simulink model "rotpentemplate"  (R2021b)
settings: Solver=VariableStepDiscrete  StartTime=0.0  StopTime=50  RelTol=1e-3  EnableMultiTasking=on
values from neighbouring files (symbols this model uses):
  adingain = [adingain 1 1 1 1 1]    [hwinit.m]    (also in theta2_bottomswing.mat = [1.276 1.276 1 1 1 1 1])
  adinoffs = [adinoffs 0 0 0 0 0]    [hwinit.m]    (also in theta2_bottomswing.mat = [-3.773 -1.223 0 0 0 0 0])
  daoutgain = 1*[-6]    [hwinit.m]    (also in theta2_bottomswing.mat = -6)
  daoutoffs = [0.00]    [hwinit.m]    (also in theta2_bottomswing.mat = 0)
  h = 0.01    [hwinit.m]    (also in mpc_controller.m = zeros(dim.nx+dim.nu, 1); theta2_bottomswing.mat = 0.05)
  K_lqr = [K_lqr, 0, 0]    [mpc_controller.m]
  model_matrices = buildmatrices(xr, model_mpc, constraint, penalty, terminal)    [mpc_controller.m]
  sys_dis = c2d(sys_ct, h)    [mpc_controller.m]
  xr = xur(1:dim.nx)    [mpc_controller.m]
undefined symbols (not defined in the file or in its folder): DiscIntNeverNeededParam, Discrete, model_mpc, Time
libraries: simulink x11, ctrlSharedLib x5, simulink_extras x1
settings Model: Creator=rbabuska  LastModifiedBy=ebonello
settings SolverCC: AlgebraicLoopSolver=TrustRegion
settings DataIOCC: LimitDataPoints=on  SaveFormat=Array  ReturnWorkspaceOutputs=off  SignalLoggingName=sigsOut
settings OptimizationCC: BooleanDataType=off  ExpressionDepthLimit=2147483647  InitFltsAndDblsToZero=on  LifeSpan=inf
settings DebuggingCC: SaveWithParameterizedLinksMsg=none  SignalResolutionControl=TryResolveAllWithWarning  MultiTaskDSMMsg=warning  MultiTaskCondExecSysMsg=none  AllowSymbolicDim=off  StateNameClashWarn=warning  SFUnexpectedBacktrackingDiag=warning  SFNoUnconditionalDefaultTransitionDiag=warning  SFExecutionAtInitializationDiag=none  ArithmeticOperatorsInVariantConditions=warning
settings HardwareCC: ProdBitPerPointer=32  ProdBitPerSizeT=32  ProdBitPerPtrDiffT=32  ProdLargestAtomicFloat=None  ProdIntDivRoundTo=Undefined  ProdEndianess=Unspecified  ProdWordSize=32  ProdHWDeviceType=32-bit Generic  TargetUnknown=on
settings ModelReferenceCC: PropagateSignalLabelsOutOfModel=off
settings SFSimCC: SimUseLocalCustomCode=off  CustomCodeUndefinedFunction=UseInterfaceOnly
settings RTWCC: RTWUseLocalCustomCode=off
settings CodeAppCC: StateflowObjectComments=on
settings GRTTargetCC: TargetFcnLib=ansi_tfl_tmw.mat  TargetLangStandard=C89/C90 (ANSI)  CombineOutputUpdateFcns=off  GRTInterface=on
settings ConfigComp: CovMetricSettings=dw  CovSaveCumulativeToWorkspaceVar=on  CovSaveSingleToWorkspaceVar=on  CovExternalEMLEnable=off

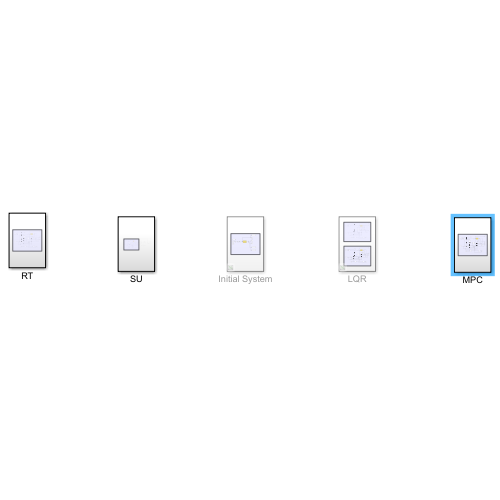
[thumbnail: Simulink's stored preview of the top-level diagram]
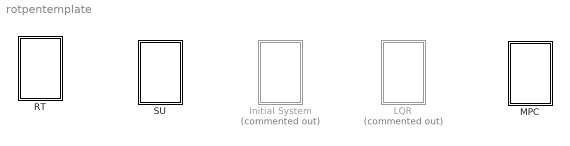
== system rotpentemplate ==
  Initial System : Subsystem  Commented=on
  LQR : Subsystem  Commented=on
  MPC : Subsystem
  RT : Subsystem
  SU : Subsystem

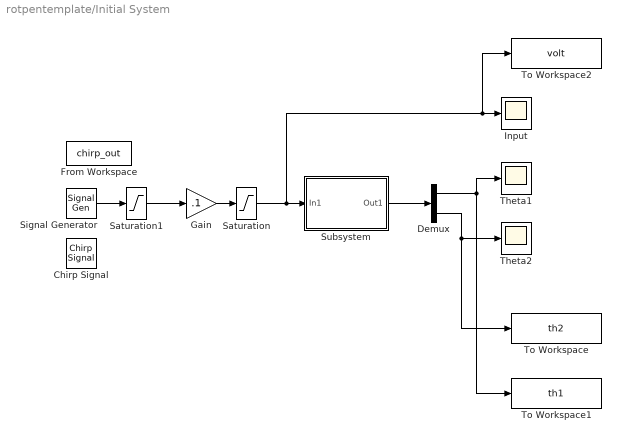
== system rotpentemplate/Initial System ==
  Chirp Signal : simulink/Sources/Chirp Signal  f1=2  T=45  f2=6
  Demux : Demux  Outputs=2
  From Workspace : FromWorkspace  VariableName=chirp_out  SampleTime=h
  Gain : Gain  Gain=.1
  Input : Scope
  Saturation : Saturate  UpperLimit=1  LowerLimit=-1
  Saturation1 : Saturate  UpperLimit=1  LowerLimit=0
  Signal Generator : SignalGenerator  WaveForm=square  Frequency=0.5
  Subsystem : Subsystem
      mask Display: disp('Rotational\nPendulum')
  Theta1 : Scope
  Theta2 : Scope
  To Workspace : ToWorkspace  VariableName=th2  SaveFormat=Timeseries  SampleTime=-1
  To Workspace1 : ToWorkspace  VariableName=th1  SaveFormat=Timeseries  SampleTime=-1
  To Workspace2 : ToWorkspace  VariableName=volt  SaveFormat=Timeseries  SampleTime=-1
  wires:
  Demux/2 -> To Workspace/1, Theta2/1
  Demux/1 -> To Workspace1/1, Theta1/1
  Subsystem/1(Out1) -> Demux/1
  Gain/1 -> Saturation/1
  Saturation/1 -> Subsystem/1(In1), To Workspace2/1, Input/1
  Signal Generator/1 -> Saturation1/1
  Saturation1/1 -> Gain/1

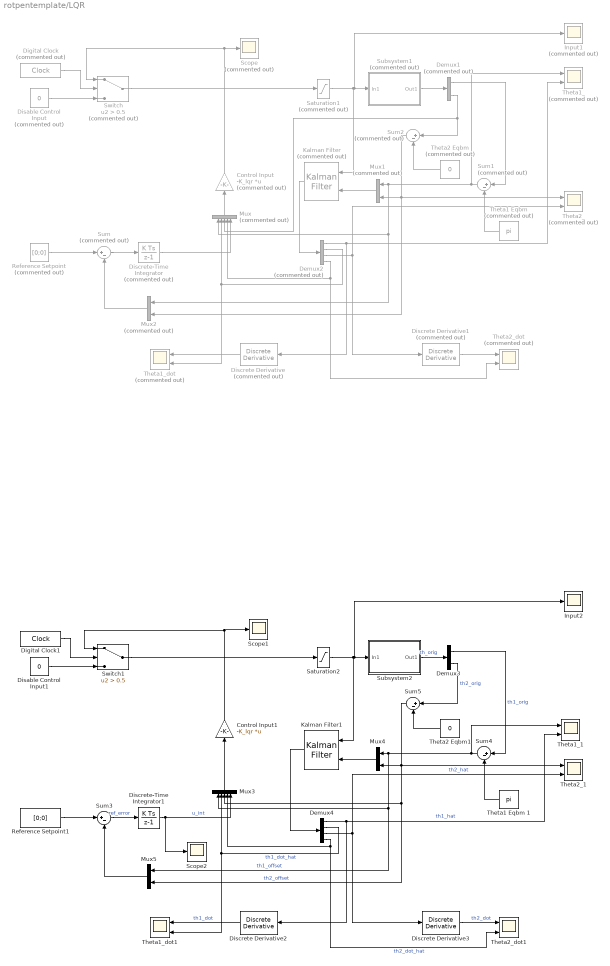
== system rotpentemplate/LQR ==
  Control Input : Gain  Commented=on  Gain=-K_lqr  Multiplication=Matrix(K*u)
  Control Input1 : Gain  Gain=-K_lqr  Multiplication=Matrix(K*u)
  Demux1 : Demux  Commented=on  Outputs=2
  Demux2 : Demux  Commented=on
  Demux3 : Demux  Outputs=2
  Demux4 : Demux
  Digital Clock : DigitalClock  Commented=on  SampleTime=h
  Digital Clock1 : DigitalClock  SampleTime=h
  Disable Control Input : Constant  Commented=on  Value=0  SampleTime=-1
  Disable Control Input1 : Constant  Value=0  SampleTime=-1
  Discrete Derivative : simulink/Discrete/Discrete Derivative  Commented=on  gainval=1.0  ICPrevScaledInput=0.0  OutMin=[]  OutMax=[]  OutDataType=fixdt(1, 16)  OutScaling=2^-10  DoSatur=off
  Discrete Derivative1 : simulink/Discrete/Discrete Derivative  Commented=on  gainval=1.0  ICPrevScaledInput=0.0  OutMin=[]  OutMax=[]  OutDataType=fixdt(1, 16)  OutScaling=2^-10  DoSatur=off
  Discrete Derivative2 : simulink/Discrete/Discrete Derivative  gainval=1.0  ICPrevScaledInput=0.0  OutMin=[]  OutMax=[]  OutDataType=fixdt(1, 16)  OutScaling=2^-10  DoSatur=off
  Discrete Derivative3 : simulink/Discrete/Discrete Derivative  gainval=1.0  ICPrevScaledInput=0.0  OutMin=[]  OutMax=[]  OutDataType=fixdt(1, 16)  OutScaling=2^-10  DoSatur=off
  Discrete-Time Integrator : DiscreteIntegrator  Commented=on  SampleTime=h  ICPrevOutput=DiscIntNeverNeededParam  ICPrevScaledInput=DiscIntNeverNeededParam
  Discrete-Time Integrator1 : DiscreteIntegrator  SampleTime=h  ICPrevOutput=DiscIntNeverNeededParam  ICPrevScaledInput=DiscIntNeverNeededParam
  Input1 : Scope  Commented=on
  Input2 : Scope
  Kalman Filter : ctrlSharedLib/Kalman Filter  Commented=on  TimeDomain=Discrete-Time  UseCurrentEstimator=on  ModelSource=Individual A, B, C, D matrices  ModelSourceVariable=ss(0.95,1,1,0,1)  A=sys_dis.A  B=sys_dis.B  C=sys_dis.C  D=sys_dis.D  NumberOfStates=1  NumberOfInputs=1  NumberOfOutputs=1  InitialEstimateSource=Dialog  X0=0  P0=10  UseK=off  UseGH=off  NumberOfProcessNoiseInputs=1  G=1  TimeInvariantG=on  H=0  TimeInvariantH=on  Q=diag([0.1^2 0.1^2 0.01^2 0.001^2])  TimeInvariantQ=on  R=diag([0.01^2 0.05^2])  TimeInvariantR=on  N=0  TimeInvariantN=on  AddInputPort=on  AddEnablePort=off  OutputEstimatedY=off  OutputP=off  Ts=-1
  Kalman Filter1 : ctrlSharedLib/Kalman Filter  TimeDomain=Discrete-Time  UseCurrentEstimator=on  ModelSource=Individual A, B, C, D matrices  ModelSourceVariable=ss(0.95,1,1,0,1)  A=sys_dis.A  B=sys_dis.B  C=sys_dis.C  D=sys_dis.D  NumberOfStates=1  NumberOfInputs=1  NumberOfOutputs=1  InitialEstimateSource=Dialog  X0=0  P0=10  UseK=off  UseGH=off  NumberOfProcessNoiseInputs=1  G=1  TimeInvariantG=on  H=0  TimeInvariantH=on  Q=diag([0.1^2 0.1^2 0.01^2 0.001^2])  TimeInvariantQ=on  R=diag([0.01^2 0.05^2])  TimeInvariantR=on  N=0  TimeInvariantN=on  AddInputPort=on  AddEnablePort=off  OutputEstimatedY=off  OutputP=off  Ts=-1
  Mux : Mux  Commented=on  Inputs=5
  Mux1 : Mux  Commented=on  Inputs=2
  Mux2 : Mux  Commented=on  Inputs=2
  Mux3 : Mux  Inputs=5
  Mux4 : Mux  Inputs=2
  Mux5 : Mux  Inputs=2
  Reference Setpoint : Constant  Commented=on  Value=[0;0]  SampleTime=-1
  Reference Setpoint1 : Constant  Value=[0;0]  SampleTime=-1
  Saturation1 : Saturate  Commented=on  UpperLimit=1  LowerLimit=-1
  Saturation2 : Saturate  UpperLimit=1  LowerLimit=-1
  Scope : Scope  Commented=on
  Scope1 : Scope
  Scope2 : Scope
  Subsystem1 : Subsystem  Commented=on
      mask Display: disp('Rotational\nPendulum')
  Subsystem2 : Subsystem
      mask Display: disp('Rotational\nPendulum')
  Sum : Sum  Commented=on  Inputs=|+-
  Sum1 : Sum  Commented=on  Inputs=|+-
  Sum2 : Sum  Commented=on  Inputs=|+-
  Sum3 : Sum  Inputs=|+-
  Sum4 : Sum  Inputs=|+-
  Sum5 : Sum  Inputs=|+-
  Switch : Switch  Commented=on  Criteria=u2 > Threshold  Threshold=0.5
  Switch1 : Switch  Criteria=u2 > Threshold  Threshold=0.5
  "Theta1 Eqbm " : Constant  Commented=on  Value=pi  SampleTime=-1
  Theta1 Eqbm 1 : Constant  Value=pi  SampleTime=-1
  Theta1_ : Scope  Commented=on  NumInputPorts=2
  Theta1_1 : Scope  NumInputPorts=2
  Theta1_dot : Scope  Commented=on  NumInputPorts=2
  Theta1_dot1 : Scope  NumInputPorts=2
  Theta2 Eqbm : Constant  Commented=on  Value=0  SampleTime=-1
  Theta2 Eqbm1 : Constant  Value=0  SampleTime=-1
  Theta2_ : Scope  Commented=on  NumInputPorts=2
  Theta2_1 : Scope  NumInputPorts=2
  Theta2_dot : Scope  Commented=on  NumInputPorts=2
  Theta2_dot1 : Scope  NumInputPorts=2
  wires:
  Demux2/3 -> Theta2_/2, Discrete Derivative1/1
  Demux1/2 -> Sum2/1, Mux/3
  Demux1/1 -> Sum1/1
  Switch/1 -> Saturation1/1
  Demux2/2 -> Theta1_dot/2, Mux/2
  Discrete Derivative1/1 -> Theta2_dot/1
  Mux/1 -> Control Input/1
  Sum/1 -> Discrete-Time Integrator/1
  Demux2/4 -> Theta2_dot/2, Mux/4
  Theta2 Eqbm/1 -> Sum2/2
  Demux2/1 -> Theta1_/2, Discrete Derivative/1
  Digital Clock/1 -> Switch/2
  Sum1/1 -> Mux2/1, Mux/1, Mux1/1, Theta1_/1
  "Theta1 Eqbm "/1 -> Sum1/2
  Disable Control Input/1 -> Switch/3
  Discrete Derivative/1 -> Theta1_dot/1
  Mux1/1 -> Kalman Filter/2
  Control Input/1 -> Scope/1, Switch/1
  Kalman Filter/1 -> Demux2/1
  Reference Setpoint/1 -> Sum/1
  Mux2/1 -> Sum/2
  Sum2/1 -> Mux1/2, Mux2/2, Theta2_/1
  Subsystem1/1(Out1) -> Demux1/1
  Saturation1/1 -> Subsystem1/1(In1), Input1/1, Kalman Filter/1
  Discrete-Time Integrator/1 -> Mux/5
  Switch1/1 -> Saturation2/1
  Discrete Derivative3/1 -> Theta2_dot1/1  "th2_dot"
  Digital Clock1/1 -> Switch1/2
  Subsystem2/1(Out1) -> Demux3/1  "th_orig"
  Sum5/1 -> Mux4/2, Mux3/3, Mux5/2, Theta2_1/1  "th2_offset"
  Demux4/3 -> Theta2_1/2, Discrete Derivative3/1  "th2_hat"
  Demux4/1 -> Theta1_1/2, Discrete Derivative2/1  "th1_hat"
  Disable Control Input1/1 -> Switch1/3
  Kalman Filter1/1 -> Demux4/1
  Sum3/1 -> Discrete-Time Integrator1/1  "ref_error"
  Discrete-Time Integrator1/1 -> Scope2/1, Mux3/5  "u_int"
  Theta1 Eqbm 1/1 -> Sum4/2
  Demux3/2 -> Sum5/1  "th2_orig"
  Mux3/1 -> Control Input1/1
  Demux4/2 -> Theta1_dot1/2, Mux3/2  "th1_dot_hat"
  Reference Setpoint1/1 -> Sum3/1
  Discrete Derivative2/1 -> Theta1_dot1/1  "th1_dot"
  Mux5/1 -> Sum3/2
  Theta2 Eqbm1/1 -> Sum5/2
  Saturation2/1 -> Subsystem2/1(In1), Input2/1, Kalman Filter1/1
  Mux4/1 -> Kalman Filter1/2
  Demux3/1 -> Sum4/1  "th1_orig"
  Sum4/1 -> Mux3/1, Mux5/1, Mux4/1, Theta1_1/1  "th1_offset"
  Demux4/4 -> Theta2_dot1/2, Mux3/4  "th2_dot_hat"
  Control Input1/1 -> Scope1/1, Switch1/1

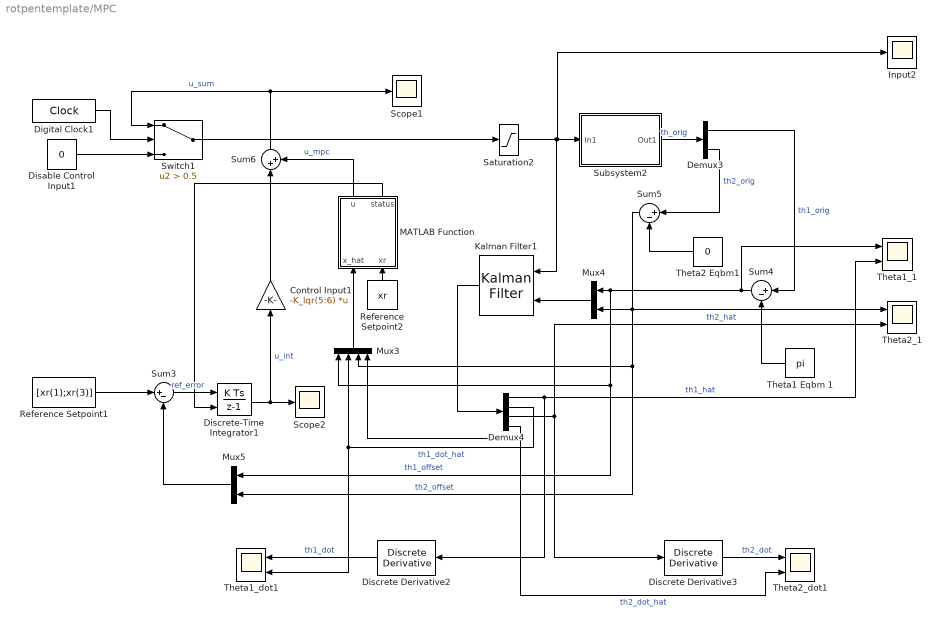
== system rotpentemplate/MPC ==
  Control Input1 : Gain  Gain=-K_lqr(5:6)  Multiplication=Matrix(K*u)
  Demux3 : Demux  Outputs=2
  Demux4 : Demux
  Digital Clock1 : DigitalClock  SampleTime=h
  Disable Control Input1 : Constant  Value=0  SampleTime=-1
  Discrete Derivative2 : simulink/Discrete/Discrete Derivative  gainval=1.0  ICPrevScaledInput=0.0  OutMin=[]  OutMax=[]  OutDataType=fixdt(1, 16)  OutScaling=2^-10  DoSatur=off
  Discrete Derivative3 : simulink/Discrete/Discrete Derivative  gainval=1.0  ICPrevScaledInput=0.0  OutMin=[]  OutMax=[]  OutDataType=fixdt(1, 16)  OutScaling=2^-10  DoSatur=off
  Discrete-Time Integrator1 : DiscreteIntegrator  ExternalReset=level  SampleTime=h  ICPrevOutput=DiscIntNeverNeededParam  ICPrevScaledInput=DiscIntNeverNeededParam
  Input2 : Scope
  Kalman Filter1 : ctrlSharedLib/Kalman Filter  TimeDomain=Discrete-Time  UseCurrentEstimator=on  ModelSource=Individual A, B, C, D matrices  ModelSourceVariable=ss(0.95,1,1,0,1)  A=sys_dis.A  B=sys_dis.B  C=sys_dis.C  D=sys_dis.D  NumberOfStates=1  NumberOfInputs=1  NumberOfOutputs=1  InitialEstimateSource=Dialog  X0=0  P0=10  UseK=off  UseGH=off  NumberOfProcessNoiseInputs=1  G=1  TimeInvariantG=on  H=0  TimeInvariantH=on  Q=diag([0.1^2 0.1^2 0.01^2 0.001^2])  TimeInvariantQ=on  R=diag([0.01^2 0.05^2])  TimeInvariantR=on  N=0  TimeInvariantN=on  AddInputPort=on  AddEnablePort=off  OutputEstimatedY=off  OutputP=off  Ts=-1
  MATLAB Function : MATLAB Function  TreatAsAtomicUnit=on
  Mux3 : Mux
  Mux4 : Mux  Inputs=2
  Mux5 : Mux  Inputs=2
  Reference Setpoint1 : Constant  Value=[xr(1);xr(3)]  SampleTime=-1
  Reference Setpoint2 : Constant  Value=xr  SampleTime=-1
  Saturation2 : Saturate  UpperLimit=1  LowerLimit=-1
  Scope1 : Scope
  Scope2 : Scope
  Subsystem2 : Subsystem
      mask Display: disp('Rotational\nPendulum')
  Sum3 : Sum  Inputs=|+-
  Sum4 : Sum  Inputs=|+-
  Sum5 : Sum  Inputs=|+-
  Sum6 : Sum  Inputs=|++
  Switch1 : Switch  Criteria=u2 > Threshold  Threshold=0.5
  Theta1 Eqbm 1 : Constant  Value=pi  SampleTime=-1
  Theta1_1 : Scope  NumInputPorts=2
  Theta1_dot1 : Scope  NumInputPorts=2
  Theta2 Eqbm1 : Constant  Value=0  SampleTime=-1
  Theta2_1 : Scope  NumInputPorts=2
  Theta2_dot1 : Scope  NumInputPorts=2
  wires:
  Mux4/1 -> Kalman Filter1/2
  Demux4/4 -> Theta2_dot1/2, Mux3/4  "th2_dot_hat"
  Sum3/1 -> Discrete-Time Integrator1/1  "ref_error"
  Sum6/1 -> Scope1/1, Switch1/1  "u_sum"
  Discrete Derivative2/1 -> Theta1_dot1/1  "th1_dot"
  Mux5/1 -> Sum3/2
  Demux3/2 -> Sum5/1  "th2_orig"
  Demux4/2 -> Theta1_dot1/2, Mux3/2  "th1_dot_hat"
  Disable Control Input1/1 -> Switch1/3
  Demux3/1 -> Sum4/1  "th1_orig"
  Reference Setpoint1/1 -> Sum3/1
  Sum4/1 -> Mux3/1, Mux5/1, Mux4/1, Theta1_1/1  "th1_offset"
  Discrete-Time Integrator1/1 -> Control Input1/1, Scope2/1  "u_int"
  MATLAB Function/1(u) -> Sum6/2  "u_mpc"
  Theta1 Eqbm 1/1 -> Sum4/2
  Saturation2/1 -> Subsystem2/1(In1), Input2/1, Kalman Filter1/1
  Demux4/1 -> Theta1_1/2, Discrete Derivative2/1  "th1_hat"
  Theta2 Eqbm1/1 -> Sum5/2
  Switch1/1 -> Saturation2/1
  Demux4/3 -> Theta2_1/2, Discrete Derivative3/1  "th2_hat"
  Digital Clock1/1 -> Switch1/2
  Mux3/1 -> MATLAB Function/1(x_hat)
  Kalman Filter1/1 -> Demux4/1
  Sum5/1 -> Mux4/2, Mux3/3, Mux5/2, Theta2_1/1  "th2_offset"
  Reference Setpoint2/1 -> MATLAB Function/2(xr)
  Control Input1/1 -> Sum6/1
  MATLAB Function/2(status) -> Discrete-Time Integrator1/2
  Subsystem2/1(Out1) -> Demux3/1  "th_orig"
  Discrete Derivative3/1 -> Theta2_dot1/1  "th2_dot"

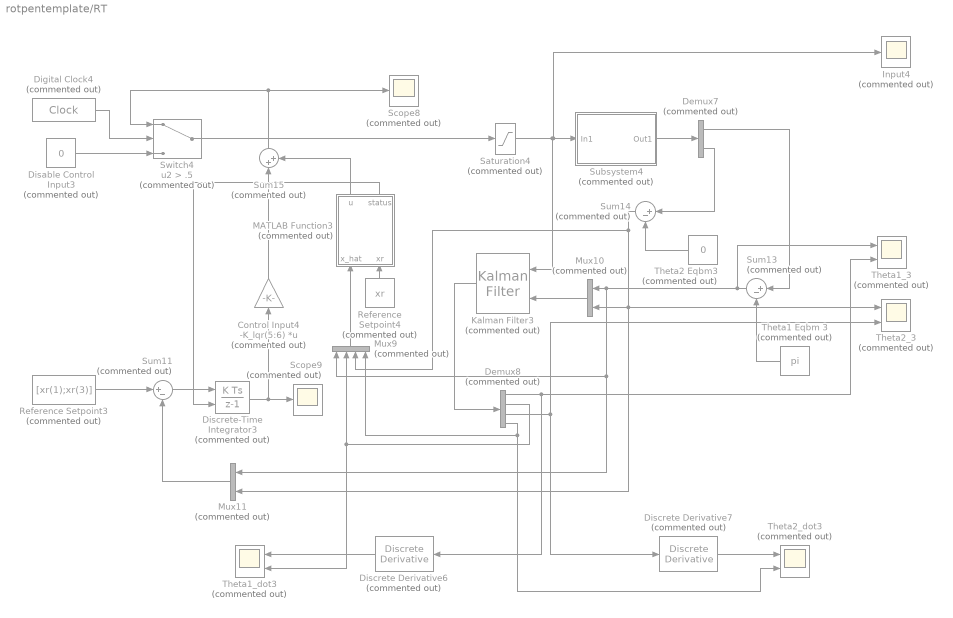
== system rotpentemplate/RT ==
  Control Input4 : Gain  Commented=on  Gain=-K_lqr(5:6)  Multiplication=Matrix(K*u)
  Demux7 : Demux  Commented=on  Outputs=2
  Demux8 : Demux  Commented=on
  Digital Clock4 : DigitalClock  Commented=on  SampleTime=h
  Disable Control Input3 : Constant  Commented=on  Value=0  SampleTime=-1
  Discrete Derivative6 : simulink/Discrete/Discrete Derivative  Commented=on  gainval=1.0  ICPrevScaledInput=0.0  OutMin=[]  OutMax=[]  OutDataType=fixdt(1, 16)  OutScaling=2^-10  DoSatur=off
  Discrete Derivative7 : simulink/Discrete/Discrete Derivative  Commented=on  gainval=1.0  ICPrevScaledInput=0.0  OutMin=[]  OutMax=[]  OutDataType=fixdt(1, 16)  OutScaling=2^-10  DoSatur=off
  Discrete-Time Integrator3 : DiscreteIntegrator  Commented=on  ExternalReset=level  SampleTime=h  ICPrevOutput=DiscIntNeverNeededParam  ICPrevScaledInput=DiscIntNeverNeededParam
  Input4 : Scope  Commented=on
  Kalman Filter3 : ctrlSharedLib/Kalman Filter  Commented=on  TimeDomain=Discrete-Time  UseCurrentEstimator=on  ModelSource=Individual A, B, C, D matrices  ModelSourceVariable=ss(0.95,1,1,0,1)  A=sys_dis.A  B=sys_dis.B  C=sys_dis.C  D=sys_dis.D  NumberOfStates=1  NumberOfInputs=1  NumberOfOutputs=1  InitialEstimateSource=Dialog  X0=0  P0=10  UseK=off  UseGH=off  NumberOfProcessNoiseInputs=1  G=1  TimeInvariantG=on  H=0  TimeInvariantH=on  Q=diag([0.1^2 0.1^2 0.01^2 0.001^2])  TimeInvariantQ=on  R=diag([0.01^2 0.05^2])  TimeInvariantR=on  N=0  TimeInvariantN=on  AddInputPort=on  AddEnablePort=off  OutputEstimatedY=off  OutputP=off  Ts=-1
  MATLAB Function3 : MATLAB Function  Commented=on  TreatAsAtomicUnit=on
  Mux10 : Mux  Commented=on  Inputs=2
  Mux11 : Mux  Commented=on  Inputs=2
  Mux9 : Mux  Commented=on
  Reference Setpoint3 : Constant  Commented=on  Value=[xr(1);xr(3)]  SampleTime=-1
  Reference Setpoint4 : Constant  Commented=on  Value=xr  SampleTime=-1
  Saturation4 : Saturate  Commented=on  UpperLimit=1  LowerLimit=-1
  Scope8 : Scope  Commented=on
  Scope9 : Scope  Commented=on
  Subsystem4 : Subsystem  Commented=on
      mask Display: disp('Rotational\nPendulum')
  Sum11 : Sum  Commented=on  Inputs=|+-
  Sum13 : Sum  Commented=on  Inputs=|+-
  Sum14 : Sum  Commented=on  Inputs=|+-
  Sum15 : Sum  Commented=on  Inputs=|++
  Switch4 : Switch  Commented=on  Criteria=u2 > Threshold  Threshold=.5
  Theta1 Eqbm 3 : Constant  Commented=on  Value=pi  SampleTime=-1
  Theta1_3 : Scope  Commented=on  NumInputPorts=2
  Theta1_dot3 : Scope  Commented=on  NumInputPorts=2
  Theta2 Eqbm3 : Constant  Commented=on  Value=0  SampleTime=-1
  Theta2_3 : Scope  Commented=on  NumInputPorts=2
  Theta2_dot3 : Scope  Commented=on  NumInputPorts=2
  wires:
  Sum14/1 -> Mux9/3, Mux10/2, Mux11/2, Theta2_3/1
  Demux8/3 -> Theta2_3/2, Discrete Derivative7/1
  Subsystem4/1(Out1) -> Demux7/1
  Discrete-Time Integrator3/1 -> Control Input4/1, Scope9/1
  Control Input4/1 -> Sum15/1
  Saturation4/1 -> Subsystem4/1(In1), Input4/1, Kalman Filter3/1
  Demux8/2 -> Theta1_dot3/2, Mux9/2
  Demux8/1 -> Theta1_3/2, Discrete Derivative6/1
  Sum11/1 -> Discrete-Time Integrator3/1
  MATLAB Function3/2(status) -> Discrete-Time Integrator3/2
  Reference Setpoint4/1 -> MATLAB Function3/2(xr)
  Kalman Filter3/1 -> Demux8/1
  Reference Setpoint3/1 -> Sum11/1
  Mux10/1 -> Kalman Filter3/2
  Sum13/1 -> Mux11/1, Mux9/1, Mux10/1, Theta1_3/1
  Mux9/1 -> MATLAB Function3/1(x_hat)
  Digital Clock4/1 -> Switch4/2
  Switch4/1 -> Saturation4/1
  Sum15/1 -> Scope8/1, Switch4/1
  Theta2 Eqbm3/1 -> Sum14/2
  Demux7/1 -> Sum13/1
  Discrete Derivative6/1 -> Theta1_dot3/1
  MATLAB Function3/1(u) -> Sum15/2
  Discrete Derivative7/1 -> Theta2_dot3/1
  Demux8/4 -> Theta2_dot3/2, Mux9/4
  Theta1 Eqbm 3/1 -> Sum13/2
  Demux7/2 -> Sum14/1
  Disable Control Input3/1 -> Switch4/3
  Mux11/1 -> Sum11/2

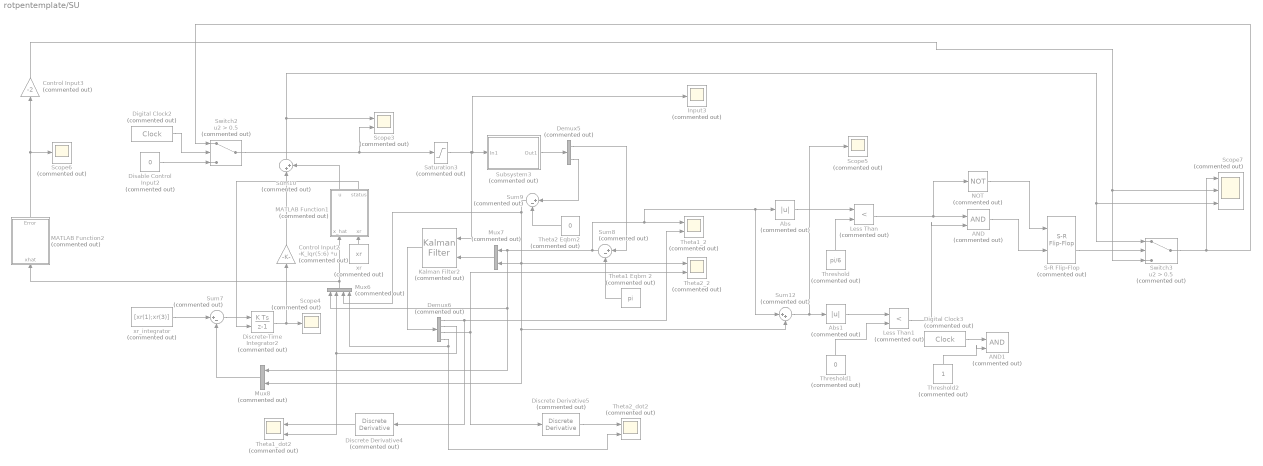
== system rotpentemplate/SU ==
  AND : Logic  Commented=on  IconShape=distinctive  AllPortsSameDT=off  OutDataTypeStr=boolean
  AND1 : Logic  Commented=on  IconShape=distinctive  AllPortsSameDT=off  OutDataTypeStr=boolean
  Abs : Abs  Commented=on
  Abs1 : Abs  Commented=on
  Control Input2 : Gain  Commented=on  Gain=-K_lqr(5:6)  Multiplication=Matrix(K*u)
  Control Input3 : Gain  Commented=on  Gain=-2
  Demux5 : Demux  Commented=on  Outputs=2
  Demux6 : Demux  Commented=on
  Digital Clock2 : DigitalClock  Commented=on  SampleTime=h
  Digital Clock3 : DigitalClock  Commented=on  SampleTime=h
  Disable Control Input2 : Constant  Commented=on  Value=0  SampleTime=-1
  Discrete Derivative4 : simulink/Discrete/Discrete Derivative  Commented=on  gainval=1.0  ICPrevScaledInput=0.0  OutMin=[]  OutMax=[]  OutDataType=fixdt(1, 16)  OutScaling=2^-10  DoSatur=off
  Discrete Derivative5 : simulink/Discrete/Discrete Derivative  Commented=on  gainval=1.0  ICPrevScaledInput=0.0  OutMin=[]  OutMax=[]  OutDataType=fixdt(1, 16)  OutScaling=2^-10  DoSatur=off
  Discrete-Time Integrator2 : DiscreteIntegrator  Commented=on  ExternalReset=level  SampleTime=h  ICPrevOutput=DiscIntNeverNeededParam  ICPrevScaledInput=DiscIntNeverNeededParam
  Input3 : Scope  Commented=on
  Kalman Filter2 : ctrlSharedLib/Kalman Filter  Commented=on  TimeDomain=Discrete-Time  UseCurrentEstimator=on  ModelSource=Individual A, B, C, D matrices  ModelSourceVariable=ss(0.95,1,1,0,1)  A=sys_dis.A  B=sys_dis.B  C=sys_dis.C  D=sys_dis.D  NumberOfStates=1  NumberOfInputs=1  NumberOfOutputs=1  InitialEstimateSource=Dialog  X0=0  P0=10  UseK=off  UseGH=off  NumberOfProcessNoiseInputs=1  G=1  TimeInvariantG=on  H=0  TimeInvariantH=on  Q=diag([0.1^2 0.1^2 0.01^2 0.001^2])  TimeInvariantQ=on  R=diag([0.01^2 0.05^2])  TimeInvariantR=on  N=0  TimeInvariantN=on  AddInputPort=on  AddEnablePort=off  OutputEstimatedY=off  OutputP=off  Ts=-1
  Less Than : RelationalOperator  Commented=on  Operator=<  OutDataTypeStr=boolean  RndMeth=Simplest
  Less Than1 : RelationalOperator  Commented=on  Operator=<  OutDataTypeStr=boolean  RndMeth=Simplest
  MATLAB Function1 : MATLAB Function  Commented=on  TreatAsAtomicUnit=on
  MATLAB Function2 : MATLAB Function  Commented=on  TreatAsAtomicUnit=on
  Mux6 : Mux  Commented=on
  Mux7 : Mux  Commented=on  Inputs=2
  Mux8 : Mux  Commented=on  Inputs=2
  NOT : Logic  Commented=on  Operator=NOT  IconShape=distinctive  AllPortsSameDT=off  OutDataTypeStr=boolean
  S-R Flip-Flop : simulink_extras/Flip Flops/S-R Flip-Flop  Commented=on  initial_condition=0
  Saturation3 : Saturate  Commented=on  UpperLimit=1  LowerLimit=-1
  Scope3 : Scope  Commented=on  NumInputPorts=2
  Scope4 : Scope  Commented=on
  Scope5 : Scope  Commented=on
  Scope6 : Scope  Commented=on
  Scope7 : Scope  Commented=on  NumInputPorts=3
  Subsystem3 : Subsystem  Commented=on
      mask Display: disp('Rotational\nPendulum')
  Sum10 : Sum  Commented=on  Inputs=|++
  Sum12 : Sum  Commented=on  Inputs=|++
  Sum7 : Sum  Commented=on  Inputs=|+-
  Sum8 : Sum  Commented=on  Inputs=|+-
  Sum9 : Sum  Commented=on  Inputs=|+-
  Switch2 : Switch  Commented=on  Criteria=u2 > Threshold  Threshold=0.5
  Switch3 : Switch  Commented=on  Criteria=u2 > Threshold  Threshold=0.5
  Theta1 Eqbm 2 : Constant  Commented=on  Value=pi  SampleTime=-1
  Theta1_2 : Scope  Commented=on  NumInputPorts=2
  Theta1_dot2 : Scope  Commented=on  NumInputPorts=2
  Theta2 Eqbm2 : Constant  Commented=on  Value=0  SampleTime=-1
  Theta2_2 : Scope  Commented=on  NumInputPorts=2
  Theta2_dot2 : Scope  Commented=on  NumInputPorts=2
  Threshold : Constant  Commented=on  Value=pi/6  SampleTime=-1
  Threshold1 : Constant  Commented=on  Value=0  SampleTime=-1
  Threshold2 : Constant  Commented=on  SampleTime=-1
  xr : Constant  Commented=on  Value=xr  SampleTime=-1
  xr_integrator : Constant  Commented=on  Value=[xr(1);xr(3)]  SampleTime=-1
  wires:
  Subsystem3/1(Out1) -> Demux5/1
  Discrete-Time Integrator2/1 -> Control Input2/1, Scope4/1
  Demux5/2 -> Sum9/1
  Control Input2/1 -> Sum10/1
  Sum9/1 -> Mux6/3, Mux8/2, Sum12/2, Theta2_2/1, Mux7/2
  Threshold1/1 -> Less Than1/2
  Abs/1 -> Less Than/1
  xr_integrator/1 -> Sum7/1
  Switch2/1 -> Saturation3/1, Scope3/2
  Sum8/1 -> Mux8/1, Mux6/1, Mux7/1, Sum12/1, Abs/1, Theta1_2/1
  Demux6/2 -> Theta1_dot2/2, Mux6/2
  Sum12/1 -> Scope5/1, Abs1/1
  Discrete Derivative4/1 -> Theta1_dot2/1
  Saturation3/1 -> Subsystem3/1(In1), Input3/1, Kalman Filter2/1
  S-R Flip-Flop/2 -> Switch3/2
  Threshold/1 -> Less Than/2
  MATLAB Function1/2(status) -> Discrete-Time Integrator2/2
  Demux6/3 -> Theta2_2/2, Discrete Derivative5/1
  Demux6/1 -> Theta1_2/2, Discrete Derivative4/1
  MATLAB Function2/1(Error) -> Control Input3/1, Scope6/1
  Demux5/1 -> Sum8/1
  Disable Control Input2/1 -> Switch2/3
  Threshold2/1 -> AND1/2
  Theta2 Eqbm2/1 -> Sum9/2
  Theta1 Eqbm 2/1 -> Sum8/2
  MATLAB Function1/1(u) -> Sum10/2
  NOT/1 -> S-R Flip-Flop/1
  Sum7/1 -> Discrete-Time Integrator2/1
  Kalman Filter2/1 -> Demux6/1
  Demux6/4 -> Theta2_dot2/2, Mux6/4
  Less Than/1 -> NOT/1, AND/1
  Switch3/1 -> Scope7/1, Switch2/1
  Mux8/1 -> Sum7/2
  Discrete Derivative5/1 -> Theta2_dot2/1
  Sum10/1 -> Scope7/3, Switch3/1, Scope3/1
  xr/1 -> MATLAB Function1/2(xr)
  Mux6/1 -> MATLAB Function2/1(xhat), MATLAB Function1/1(x_hat)
  Digital Clock2/1 -> Switch2/2
  Mux7/1 -> Kalman Filter2/2
  Less Than1/1 -> AND/2
  Digital Clock3/1 -> AND1/1
  Control Input3/1 -> Switch3/3, Scope7/2
  Abs1/1 -> Less Than1/1
  AND/1 -> S-R Flip-Flop/2

== system rotpentemplate/Initial System/Subsystem ==
  In1 : Inport
  Demux : Demux  Outputs=[2 4 1]
  RT input : Subsystem  mask{Ts=h, channels=[6 7]}
      mask prompts: Ts "Sample time [s]:"; channels "Channels to read (e.g., [6 7])"
      mask init:
      | hwinit;
      | 
      | % initialize FPGA
      | fugihandle = fugiboard('Open', 'Pendulum1');
      | fugihandle.WatchdogTimeout = 0.5;
      | fugiboard('SetParams', fugihandle);
      | fugiboard('Write', fugihandle, 0, 0, 0, 0);  % dummy write to sync interface board
      | fugiboard('Write', fugihandle, 5, 1, 0, 0);  % reset position, activate relay
      | data = fugiboard('Read', fugihandle);        % get version info from FPGA
      | % model = bitshift(data(1), -5); 
      | % version = bitand(data(1), 31);
      | % disp(sprintf('FPGA setup %d, version %d', model, version)); % for the B&P it should say 1 1, or else there is a problem
      | fugiboard('Write', fugihandle, 0, 1, 0, 0);  % end reset
      | pause(0.1);                         % give relay some time to respond
      mask Display: disp('Rotational\nPendulum')
  Out1 : Outport
  tag scope: enc=global, switch=global
  wires:
  RT input/1(Angles) -> Demux/1
  Demux/1 -> Out1/1
  Demux/2 -> [switch]
  Demux/3 -> [enc]
  In1/1 -> RT input/1(Motors)

== system rotpentemplate/LQR/Subsystem1 ==
  In1 : Inport
  Demux : Demux  Outputs=[2 4 1]
  RT input : Subsystem  mask{Ts=h, channels=[6 7]}
      mask prompts: Ts "Sample time [s]:"; channels "Channels to read (e.g., [6 7])"
      mask init: same as rotpentemplate/Initial System/Subsystem/RT input
      mask Display: disp('Rotational\nPendulum')
  Out1 : Outport
  tag scope: enc=global, switch=global
  wires:
  RT input/1(Angles) -> Demux/1
  Demux/1 -> Out1/1
  Demux/2 -> [switch]
  Demux/3 -> [enc]
  In1/1 -> RT input/1(Motors)

== system rotpentemplate/LQR/Subsystem2 ==
  In1 : Inport
  Demux : Demux  Outputs=[2 4 1]
  RT input : Subsystem  mask{Ts=h, channels=[6 7]}
      mask prompts: Ts "Sample time [s]:"; channels "Channels to read (e.g., [6 7])"
      mask init: same as rotpentemplate/Initial System/Subsystem/RT input
      mask Display: disp('Rotational\nPendulum')
  Out1 : Outport
  tag scope: enc=global, switch=global
  wires:
  RT input/1(Angles) -> Demux/1
  Demux/1 -> Out1/1
  Demux/2 -> [switch]
  Demux/3 -> [enc]
  In1/1 -> RT input/1(Motors)

== system rotpentemplate/MPC/Subsystem2 ==
  In1 : Inport
  Demux : Demux  Outputs=[2 4 1]
  RT input : Subsystem  mask{Ts=h, channels=[6 7]}
      mask prompts: Ts "Sample time [s]:"; channels "Channels to read (e.g., [6 7])"
      mask init: same as rotpentemplate/Initial System/Subsystem/RT input
      mask Display: disp('Rotational\nPendulum')
  Out1 : Outport
  tag scope: enc=global, switch=global
  wires:
  RT input/1(Angles) -> Demux/1
  Demux/1 -> Out1/1
  Demux/2 -> [switch]
  Demux/3 -> [enc]
  In1/1 -> RT input/1(Motors)

== system rotpentemplate/RT/Subsystem4 ==
  In1 : Inport
  Demux : Demux  Outputs=[2 4 1]
  RT input : Subsystem  mask{Ts=h, channels=[6 7]}
      mask prompts: Ts "Sample time [s]:"; channels "Channels to read (e.g., [6 7])"
      mask init: same as rotpentemplate/Initial System/Subsystem/RT input
      mask Display: disp('Rotational\nPendulum')
  Out1 : Outport
  tag scope: enc=global, switch=global
  wires:
  RT input/1(Angles) -> Demux/1
  Demux/1 -> Out1/1
  Demux/2 -> [switch]
  Demux/3 -> [enc]
  In1/1 -> RT input/1(Motors)

== system rotpentemplate/SU/Subsystem3 ==
  In1 : Inport
  Demux : Demux  Outputs=[2 4 1]
  RT input : Subsystem  mask{Ts=h, channels=[6 7]}
      mask prompts: Ts "Sample time [s]:"; channels "Channels to read (e.g., [6 7])"
      mask init: same as rotpentemplate/Initial System/Subsystem/RT input
      mask Display: disp('Rotational\nPendulum')
  Out1 : Outport
  tag scope: enc=global, switch=global
  wires:
  RT input/1(Angles) -> Demux/1
  Demux/1 -> Out1/1
  Demux/2 -> [switch]
  Demux/3 -> [enc]
  In1/1 -> RT input/1(Motors)

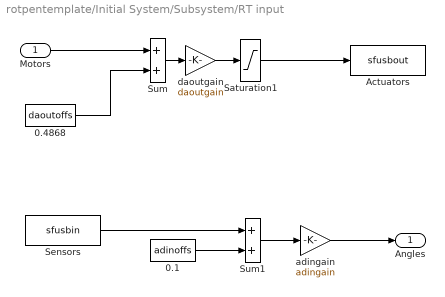
== system rotpentemplate/Initial System/Subsystem/RT input ==
  Motors : Inport
  0.1 : Constant  Value=adinoffs
  0.4868 : Constant  Value=daoutoffs
  Actuators : S-Function  FunctionName=sfusbout  Parameters=Ts, fugihandle  SFunctionDeploymentMode=off  EnableBusSupport=off
  Saturation1 : Saturate  UpperLimit=10  LowerLimit=-10
  Sensors : S-Function  FunctionName=sfusbin  Parameters=Ts, fugihandle, channels  SFunctionDeploymentMode=off  EnableBusSupport=off
  Sum : Sum  InputSameDT=on  SaturateOnIntegerOverflow=on  OutDataTypeStr=Inherit: Same as first input
  Sum1 : Sum  InputSameDT=on  SaturateOnIntegerOverflow=on  OutDataTypeStr=Inherit: Same as first input
  adingain : Gain  Gain=adingain  SaturateOnIntegerOverflow=on  OutDataTypeStr=Inherit: Same as input  ParamDataTypeStr=Inherit: Same as input
  daoutgain : Gain  Gain=daoutgain  SaturateOnIntegerOverflow=on  OutDataTypeStr=Inherit: Same as input  ParamDataTypeStr=Inherit: Same as input
  Angles : Outport
  wires:
  Sum/1 -> daoutgain/1
  0.4868/1 -> Sum/2
  Motors/1 -> Sum/1
  Sum1/1 -> adingain/1
  0.1/1 -> Sum1/2
  adingain/1 -> Angles/1
  Saturation1/1 -> Actuators/1
  daoutgain/1 -> Saturation1/1
  Sensors/1 -> Sum1/1

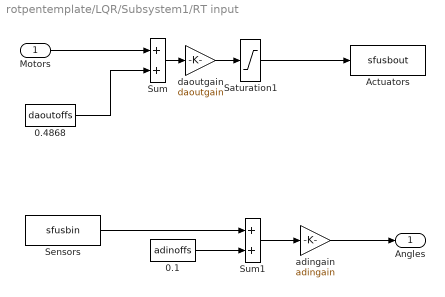
== system rotpentemplate/LQR/Subsystem1/RT input ==
  Motors : Inport
  0.1 : Constant  Value=adinoffs
  0.4868 : Constant  Value=daoutoffs
  Actuators : S-Function  FunctionName=sfusbout  Parameters=Ts, fugihandle  SFunctionDeploymentMode=off  EnableBusSupport=off
  Saturation1 : Saturate  UpperLimit=10  LowerLimit=-10
  Sensors : S-Function  FunctionName=sfusbin  Parameters=Ts, fugihandle, channels  SFunctionDeploymentMode=off  EnableBusSupport=off
  Sum : Sum  InputSameDT=on  SaturateOnIntegerOverflow=on  OutDataTypeStr=Inherit: Same as first input
  Sum1 : Sum  InputSameDT=on  SaturateOnIntegerOverflow=on  OutDataTypeStr=Inherit: Same as first input
  adingain : Gain  Gain=adingain  SaturateOnIntegerOverflow=on  OutDataTypeStr=Inherit: Same as input  ParamDataTypeStr=Inherit: Same as input
  daoutgain : Gain  Gain=daoutgain  SaturateOnIntegerOverflow=on  OutDataTypeStr=Inherit: Same as input  ParamDataTypeStr=Inherit: Same as input
  Angles : Outport
  wires:
  Sum/1 -> daoutgain/1
  0.4868/1 -> Sum/2
  Motors/1 -> Sum/1
  Sum1/1 -> adingain/1
  0.1/1 -> Sum1/2
  adingain/1 -> Angles/1
  Saturation1/1 -> Actuators/1
  daoutgain/1 -> Saturation1/1
  Sensors/1 -> Sum1/1

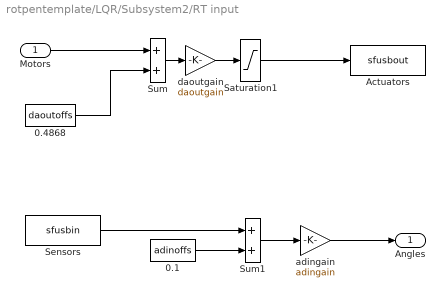
== system rotpentemplate/LQR/Subsystem2/RT input ==
  Motors : Inport
  0.1 : Constant  Value=adinoffs
  0.4868 : Constant  Value=daoutoffs
  Actuators : S-Function  FunctionName=sfusbout  Parameters=Ts, fugihandle  SFunctionDeploymentMode=off  EnableBusSupport=off
  Saturation1 : Saturate  UpperLimit=10  LowerLimit=-10
  Sensors : S-Function  FunctionName=sfusbin  Parameters=Ts, fugihandle, channels  SFunctionDeploymentMode=off  EnableBusSupport=off
  Sum : Sum  InputSameDT=on  SaturateOnIntegerOverflow=on  OutDataTypeStr=Inherit: Same as first input
  Sum1 : Sum  InputSameDT=on  SaturateOnIntegerOverflow=on  OutDataTypeStr=Inherit: Same as first input
  adingain : Gain  Gain=adingain  SaturateOnIntegerOverflow=on  OutDataTypeStr=Inherit: Same as input  ParamDataTypeStr=Inherit: Same as input
  daoutgain : Gain  Gain=daoutgain  SaturateOnIntegerOverflow=on  OutDataTypeStr=Inherit: Same as input  ParamDataTypeStr=Inherit: Same as input
  Angles : Outport
  wires:
  Sum/1 -> daoutgain/1
  0.4868/1 -> Sum/2
  Motors/1 -> Sum/1
  Sum1/1 -> adingain/1
  0.1/1 -> Sum1/2
  adingain/1 -> Angles/1
  Saturation1/1 -> Actuators/1
  daoutgain/1 -> Saturation1/1
  Sensors/1 -> Sum1/1

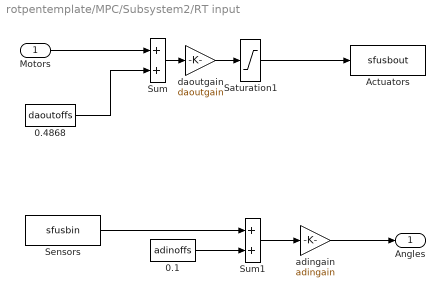
== system rotpentemplate/MPC/Subsystem2/RT input ==
  Motors : Inport
  0.1 : Constant  Value=adinoffs
  0.4868 : Constant  Value=daoutoffs
  Actuators : S-Function  FunctionName=sfusbout  Parameters=Ts, fugihandle  SFunctionDeploymentMode=off  EnableBusSupport=off
  Saturation1 : Saturate  UpperLimit=10  LowerLimit=-10
  Sensors : S-Function  FunctionName=sfusbin  Parameters=Ts, fugihandle, channels  SFunctionDeploymentMode=off  EnableBusSupport=off
  Sum : Sum  InputSameDT=on  SaturateOnIntegerOverflow=on  OutDataTypeStr=Inherit: Same as first input
  Sum1 : Sum  InputSameDT=on  SaturateOnIntegerOverflow=on  OutDataTypeStr=Inherit: Same as first input
  adingain : Gain  Gain=adingain  SaturateOnIntegerOverflow=on  OutDataTypeStr=Inherit: Same as input  ParamDataTypeStr=Inherit: Same as input
  daoutgain : Gain  Gain=daoutgain  SaturateOnIntegerOverflow=on  OutDataTypeStr=Inherit: Same as input  ParamDataTypeStr=Inherit: Same as input
  Angles : Outport
  wires:
  Sum/1 -> daoutgain/1
  0.4868/1 -> Sum/2
  Motors/1 -> Sum/1
  Sum1/1 -> adingain/1
  0.1/1 -> Sum1/2
  adingain/1 -> Angles/1
  Saturation1/1 -> Actuators/1
  daoutgain/1 -> Saturation1/1
  Sensors/1 -> Sum1/1

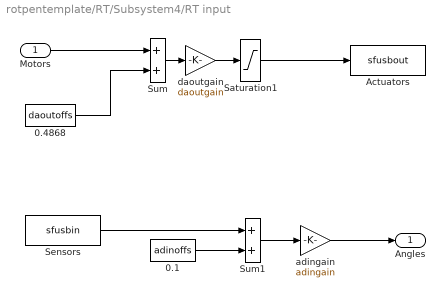
== system rotpentemplate/RT/Subsystem4/RT input ==
  Motors : Inport
  0.1 : Constant  Value=adinoffs
  0.4868 : Constant  Value=daoutoffs
  Actuators : S-Function  FunctionName=sfusbout  Parameters=Ts, fugihandle  SFunctionDeploymentMode=off  EnableBusSupport=off
  Saturation1 : Saturate  UpperLimit=10  LowerLimit=-10
  Sensors : S-Function  FunctionName=sfusbin  Parameters=Ts, fugihandle, channels  SFunctionDeploymentMode=off  EnableBusSupport=off
  Sum : Sum  InputSameDT=on  SaturateOnIntegerOverflow=on  OutDataTypeStr=Inherit: Same as first input
  Sum1 : Sum  InputSameDT=on  SaturateOnIntegerOverflow=on  OutDataTypeStr=Inherit: Same as first input
  adingain : Gain  Gain=adingain  SaturateOnIntegerOverflow=on  OutDataTypeStr=Inherit: Same as input  ParamDataTypeStr=Inherit: Same as input
  daoutgain : Gain  Gain=daoutgain  SaturateOnIntegerOverflow=on  OutDataTypeStr=Inherit: Same as input  ParamDataTypeStr=Inherit: Same as input
  Angles : Outport
  wires:
  Sum/1 -> daoutgain/1
  0.4868/1 -> Sum/2
  Motors/1 -> Sum/1
  Sum1/1 -> adingain/1
  0.1/1 -> Sum1/2
  adingain/1 -> Angles/1
  Saturation1/1 -> Actuators/1
  daoutgain/1 -> Saturation1/1
  Sensors/1 -> Sum1/1

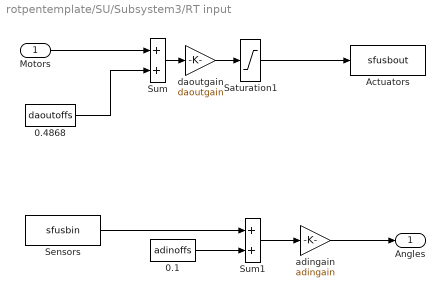
== system rotpentemplate/SU/Subsystem3/RT input ==
  Motors : Inport
  0.1 : Constant  Value=adinoffs
  0.4868 : Constant  Value=daoutoffs
  Actuators : S-Function  FunctionName=sfusbout  Parameters=Ts, fugihandle  SFunctionDeploymentMode=off  EnableBusSupport=off
  Saturation1 : Saturate  UpperLimit=10  LowerLimit=-10
  Sensors : S-Function  FunctionName=sfusbin  Parameters=Ts, fugihandle, channels  SFunctionDeploymentMode=off  EnableBusSupport=off
  Sum : Sum  InputSameDT=on  SaturateOnIntegerOverflow=on  OutDataTypeStr=Inherit: Same as first input
  Sum1 : Sum  InputSameDT=on  SaturateOnIntegerOverflow=on  OutDataTypeStr=Inherit: Same as first input
  adingain : Gain  Gain=adingain  SaturateOnIntegerOverflow=on  OutDataTypeStr=Inherit: Same as input  ParamDataTypeStr=Inherit: Same as input
  daoutgain : Gain  Gain=daoutgain  SaturateOnIntegerOverflow=on  OutDataTypeStr=Inherit: Same as input  ParamDataTypeStr=Inherit: Same as input
  Angles : Outport
  wires:
  Sum/1 -> daoutgain/1
  0.4868/1 -> Sum/2
  Motors/1 -> Sum/1
  Sum1/1 -> adingain/1
  0.1/1 -> Sum1/2
  adingain/1 -> Angles/1
  Saturation1/1 -> Actuators/1
  daoutgain/1 -> Saturation1/1
  Sensors/1 -> Sum1/1

== matlab function rotpentemplate/SU/MATLAB Function1 ==
  data: x_hat input; xr input; u output; model_mpc parameter; model_matrices parameter; status output
function [u, status] = fcn(x_hat, xr, model_mpc, model_matrices)

    ref = [repmat([xr;0], model_mpc.N, 1); xr];
    x0 = x_hat(1:4);
    dist = 0;

    % Get sizes.
    [numx, numu] = size(model_mpc.B);
    N = model_mpc.N;
    numVar = N*(numx + numu) + numx;
    
    % Update initial condition.
    model_matrices.lb(1:numx) = x0;
    model_matrices.ub(1:numx) = x0; % Fix x0 so that it optimizes u only and x is changed by system dynamics
    
    % Get vectors to extract x and u from big column vector.
    allinds = mod(0:numVar - 1, numx + numu);
    xinds = allinds < numx;
    uinds = allinds >= numx;
    
    Options = optimoptions('quadprog', 'Algorithm', 'active-set', 'Display', 'none');
    
    % Initialization
    %X = zeros(4, numVar);
    status = 0;
%     Uk = zeros(numu, N);

    H = model_matrices.H;
    f = model_matrices.f' - ref'*model_matrices.H;  %define cost function
    A = model_matrices.Alt;
    b =  model_matrices.blt;
    Aeq = model_matrices.Aeq;
    beq = model_matrices.beq - dist;
    [X, ~, status] = quadprog(H,f, A, b, Aeq, beq, model_matrices.lb, model_matrices.ub, [x_hat(1:4); zeros(numVar-numx, 1)], Options);
    
%     X(uinds)
    if status == 1
%         FVAL = 0.5*(X-ref)'*model_matrices.H*(X-ref) + model_matrices.f'*(X-ref);
%         Xk = reshape(X(xinds), numx, N + 1);
%         Uk = reshape(X(uinds), numu, N)
        u = X(5)
        status = 0;
    else
%         FVAL = 0;
%         Xk = 0;
        u = 0;
        status = 1;
        disp("Exceeding constraints");
    end

    
    
end

== matlab function rotpentemplate/MPC/MATLAB Function ==
  data: x_hat input; xr input; u output; model_mpc parameter; model_matrices parameter; status output
function [u, status] = fcn(x_hat, xr, model_mpc, model_matrices)
% function [u, status] = fcn(x_hat, xr, model_mpc, model_matrices)

    ref = [repmat([xr;0], model_mpc.N, 1); xr];
    x0 = x_hat(1:4);
    dist = 0;

    % Get sizes.
    [numx, numu] = size(model_mpc.B);
    N = model_mpc.N;
    numVar = N*(numx + numu) + numx;
    
    % Update initial condition.
    model_matrices.lb(1:numx) = x0;
    model_matrices.ub(1:numx) = x0; % Fix x0 so that it optimizes u only and x is changed by system dynamics
    
    % Get vectors to extract x and u from big column vector.
    allinds = mod(0:numVar - 1, numx + numu);
    xinds = allinds < numx;
    uinds = allinds >= numx;
    
    Options = optimoptions('quadprog', 'Algorithm', 'active-set', 'Display', 'none');
    
    % Initialization
    %X = zeros(4, numVar);
    status = 0;
%     Uk = zeros(numu, N);

    H = model_matrices.H;
    f = model_matrices.f' - ref'*model_matrices.H;  %define cost function
    A = model_matrices.Alt;
    b =  model_matrices.blt;
    Aeq = model_matrices.Aeq;
    beq = model_matrices.beq - dist;
    [X, ~, status] = quadprog(H,f, A, b, Aeq, beq, model_matrices.lb, model_matrices.ub, [x_hat(1:4); zeros(numVar-numx, 1)], Options);
    
%     X(uinds)
    if status == 1
%         FVAL = 0.5*(X-ref)'*model_matrices.H*(X-ref) + model_matrices.f'*(X-ref);
%         Xk = reshape(X(xinds), numx, N + 1);
%         Uk = reshape(X(uinds), numu, N)
        u = X(5)
        status = 0;
    else
        u = 0;
        status = 1;
        disp("Exceeding constraints");
    end
    
end

== matlab function rotpentemplate/SU/MATLAB Function2 ==
  data: xhat input; Error output
function Error = fcn(xhat)

T_act = (213292372244054040598424886087334197*xhat(2)^2)/20769187434139310514121985316880384000 + (309892187797196324531168444732106773*(xhat(2) ...
    + xhat(4))^2)/2076918743413931051412198531688038400000 + (33032383440296366935060501024173531*cos(xhat(3))*xhat(2)*(xhat(2) + xhat(4)))/103845937170696552570609926584401920000;
    
U_act = - (14595435424578591487917*cos(xhat(1)))/72057594037927936000000 - (23546223465226859843811*cos(xhat(1) + xhat(3)))/720575940379279360000000;

T_des = 0;

U_des = 0.2352;

Error = (T_des + U_des) - (T_act + U_act);

end

== matlab function rotpentemplate/RT/MATLAB Function3 ==
  data: x_hat input; xr input; u output; model_mpc parameter; model_matrices parameter; status output
function [u, status] = fcn(x_hat, xr, model_mpc, model_matrices)


x_ref = pi/6;
yref = [-x_ref; x_ref];
d_hat = 0;

    yref = sin(t)

    xr

    

    xr = targetSelector(model_mpc, Z.lqr, dim, d_hat, yref);
    model_matrices = buildmatrices(xr, model_mpc, constraint, penalty, terminal);





    ref = [repmat([xr;0], model_mpc.N, 1); xr];
    x0 = x_hat(1:4);
    dist = 0;

    % Get sizes.
    [numx, numu] = size(model_mpc.B);
    N = model_mpc.N;
    numVar = N*(numx + numu) + numx;
    
    % Update initial condition.
    model_matrices.lb(1:numx) = x0;
    model_matrices.ub(1:numx) = x0; % Fix x0 so that it optimizes u only and x is changed by system dynamics
    
    % Get vectors to extract x and u from big column vector.
    allinds = mod(0:numVar - 1, numx + numu);
    xinds = allinds < numx;
    uinds = allinds >= numx;
    
    Options = optimoptions('quadprog', 'Algorithm', 'active-set', 'Display', 'none');
    
    % Initialization
    %X = zeros(4, numVar);
    status = 0;
%     Uk = zeros(numu, N);

    H = model_matrices.H;
    f = model_matrices.f' - ref'*model_matrices.H;  %define cost function
    A = model_matrices.Alt;
    b =  model_matrices.blt;
    Aeq = model_matrices.Aeq;
    beq = model_matrices.beq - dist;
    [X, ~, status] = quadprog(H,f, A, b, Aeq, beq, model_matrices.lb, model_matrices.ub, [x_hat(1:4); zeros(numVar-numx, 1)], Options);
    
%     X(uinds)
    if status == 1
%         FVAL = 0.5*(X-ref)'*model_matrices.H*(X-ref) + model_matrices.f'*(X-ref);
%         Xk = reshape(X(xinds), numx, N + 1);
%         Uk = reshape(X(uinds), numu, N)
        u = X(5)
        status = 0;
    else
%         FVAL = 0;
%         Xk = 0;
        u = 0;
        status = 1;
        disp("Exceeding constraints");
    end

    
    
end
